simulink model "floating_control"  (Simulink 3.00)
libraries: mathlib x6, execlib x2, reglib x2, analoglib x1, arclib x1

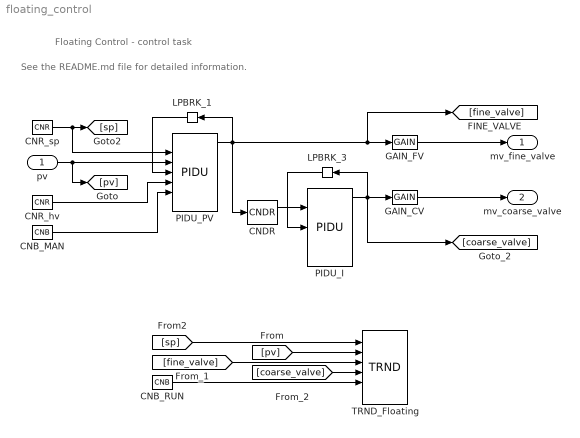
== system floating_control ==
  note: See the README.md file for detailed information.
  note: Floating Control - control task
  pv : Inport  Port=1
  CNB_MAN : mathlib/CNB  YCN=off
  CNB_RUN : mathlib/CNB  YCN=on
  CNDR : analoglib/CNDR  n=4  SATF=off  up=[ 0.0, 0.25, 0.75, 1.0]  yp=[ -0.25, 0.0, 0.0, 0.25]
  CNR_hv : mathlib/CNR  ycn=0.1
  CNR_sp : mathlib/CNR  ycn=0
  GAIN_CV : mathlib/GAIN  k=0.8
  GAIN_FV : mathlib/GAIN  k=0.2
  LPBRK_1 : execlib/LPBRK  Orientation=left
  LPBRK_3 : execlib/LPBRK  Orientation=left
  PIDU_I : reglib/PIDU  irtype=2: I  RACT=off  k=1.0  ti=20  td=1  nd=10  b=1  c=0  tt=1  hilim=1  lolim=0  dz=0  icotype=1: Analog
  PIDU_PV : reglib/PIDU  irtype=7: PID  RACT=off  k=2  ti=4  td=1  nd=10  b=1  c=0  tt=1  hilim=1  lolim=0  dz=0  icotype=1: Analog
  TRND_Floating : arclib/TRND  n=4  l=1000  btype=8: Double  ptype1=1: Store  ptype2=1: Store  ptype3=1: Store  ptype4=1: Store  pfac=1  afac=0  arc=0  id=1  Title=Trend Title  timesrc=1
  mv_fine_valve : Outport  Port=1
  mv_coarse_valve : Outport  Port=2
  wires:
  CNB_MAN/1 -> PIDU_PV/6
  CNB_RUN/1 -> TRND_Floating/5
  CNDR/1 -> PIDU_I/2
  CNR_hv/1 -> PIDU_PV/5
  CNR_sp/1 -> [sp], PIDU_PV/2
  [pv] -> TRND_Floating/2
  [sp] -> TRND_Floating/1
  [fine_valve] -> TRND_Floating/3
  [coarse_valve] -> TRND_Floating/4
  GAIN_CV/1 -> mv_coarse_valve/1
  GAIN_FV/1 -> mv_fine_valve/1
  LPBRK_1/1 -> PIDU_PV/4
  LPBRK_3/1 -> PIDU_I/4
  PIDU_I/1 -> GAIN_CV/1, [coarse_valve], LPBRK_3/1
  PIDU_PV/1 -> CNDR/1, LPBRK_1/1, [fine_valve], GAIN_FV/1
  pv/1 -> [pv], PIDU_PV/3
